simulink model "QuadcopterModel"  (R2018a)
settings: Solver=ode1  StartTime=0.0  StopTime=10.0  FixedStep=T  RelTol=1e-3  EnableMultiTasking=on
undefined symbols (not defined in the file): g, I, I_add, I_add_time, K, L, m, m_add, m_add_time, omega0, Phi0, Psi0, rho_ge, Rp, T_add, T_add_time, Theta0, V0, X0, Xmax, Xmin, Zg
libraries: UAV_Control x3
settings Model: Creator=ahmad  LastModifiedBy=Ahmad
settings OptimizationCC: LifeSpan=inf
settings DebuggingCC: SFUnexpectedBacktrackingDiag=warning  SFNoUnconditionalDefaultTransitionDiag=warning  SFExecutionAtInitializationDiag=none
settings CodeAppCC: StateflowObjectComments=on
settings GRTTargetCC: TargetLangStandard=C89/C90 (ANSI)  GeneratePreprocessorConditionals=Disable all
settings ConfigComp: CovMetricSettings=dw  CovHtmlReporting=on  CovSaveCumulativeToWorkspaceVar=on  CovSaveSingleToWorkspaceVar=on  CovExternalEMLEnable=off

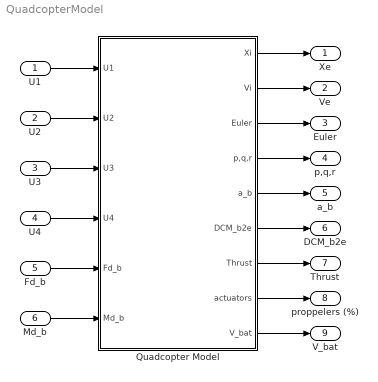
== system QuadcopterModel ==
  U1 : Inport
  U2 : Inport  Port=2
  U3 : Inport  Port=3
  U4 : Inport  Port=4
  Fd_b : Inport  Port=5
  Md_b : Inport  Port=6
  Quadcopter Model : Subsystem  mask(QuadcopterModel){}
      mask Display:
      | port_label('input',1,'U1','texmode','on')
      | port_label('input',2,'U2','texmode','on')
      | port_label('input',3,'U3','texmode','on')
      | port_label('input',4,'U4','texmode','on')
      | port_label('input',5,'Fd_b','texmode','on')
      | port_label('input',6,'Md_b','texmode','on')
      | 
      | port_label('output',1,'Xe (m)','texmode','on')
      | port_label('output',2,'Ve (m/s)','texmode','on')
      | port_label('output',3,'\phi \theta \psi (rad/s)','texmode','on')
      | port_label('output',4,'p,q,r (rad/s^2)','texmode','on')
      | port_label('output',5,'a_b (m/s^2)','texmode','on')
      | port_label('output',6,'DCM_{b2e}','texmode','on')
      | port_label('output',7,'Thrust (N)','texmode','on')
      | port_label('output',8,'proppelers (%)','texmode','on')
      | port_label('output',9,'V_{bat}','texmode','on')
  Xe : Outport
  Ve : Outport  Port=2
  "Euler " : Outport  Port=3
  p,q,r : Outport  Port=4
  a_b : Outport  Port=5
  DCM_b2e : Outport  Port=6
  Thrust : Outport  Port=7
  proppelers (%) : Outport  Port=8
  V_bat : Outport  Port=9
  wires:
  U1/1 -> Quadcopter Model/1(U1)
  U2/1 -> Quadcopter Model/2(U2)
  U3/1 -> Quadcopter Model/3(U3)
  Quadcopter Model/1(Xi) -> Xe/1
  Quadcopter Model/2(Vi) -> Ve/1
  Quadcopter Model/3("Euler ") -> "Euler "/1
  Quadcopter Model/4(p,q,r) -> p,q,r/1
  U4/1 -> Quadcopter Model/4(U4)
  Quadcopter Model/7(Thrust) -> Thrust/1
  Fd_b/1 -> Quadcopter Model/5(Fd_b)
  Quadcopter Model/8(actuators) -> proppelers (%)/1
  Quadcopter Model/6(DCM_b2e) -> DCM_b2e/1
  Quadcopter Model/5(a_b) -> a_b/1
  Md_b/1 -> Quadcopter Model/6(Md_b)
  Quadcopter Model/9(V_bat) -> V_bat/1

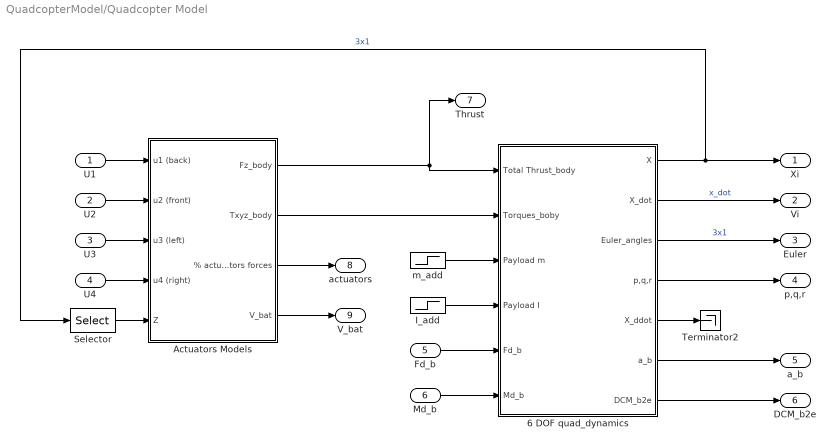
== system QuadcopterModel/Quadcopter Model ==
  U1 : Inport
  U2 : Inport  Port=2
  U3 : Inport  Port=3
  U4 : Inport  Port=4
  Fd_b : Inport  Port=5
  Md_b : Inport  Port=6
  6 DOF quad_dynamics : Subsystem
  Actuators Models : Subsystem
  I_add : Step  Time=I_add_time  After=I_add  SampleTime=0
  Selector : Selector  InputPortWidth=3  IndexOptions=Index vector (dialog)  Indices=3  OutputSizes=1
  Terminator2 : Terminator
  m_add : Step  Time=m_add_time  After=m_add  SampleTime=0
  Xi : Outport
  Vi : Outport  Port=2
  "Euler " : Outport  Port=3
  p,q,r : Outport  Port=4
  a_b : Outport  Port=5
  DCM_b2e : Outport  Port=6
  Thrust : Outport  Port=7
  actuators : Outport  Port=8
  V_bat : Outport  Port=9
  wires:
  6 DOF quad_dynamics/3(Euler_angles) -> "Euler "/1  "3x1"
  6 DOF quad_dynamics/2(X_dot) -> Vi/1  "x_dot"
  6 DOF quad_dynamics/4(p,q,r) -> p,q,r/1
  U2/1 -> Actuators Models/2(u2 (front))
  U3/1 -> Actuators Models/3(u3 (left))
  U4/1 -> Actuators Models/4(u4 (right))
  Actuators Models/3(% actuators forces) -> actuators/1
  6 DOF quad_dynamics/6(a_b) -> a_b/1
  6 DOF quad_dynamics/1(X) -> Selector/1, Xi/1  "3x1"
  U1/1 -> Actuators Models/1(u1 (back))
  Actuators Models/1(Fz_body) -> 6 DOF quad_dynamics/1("Total Thrust_body "), Thrust/1
  Actuators Models/2(Txyz_body) -> 6 DOF quad_dynamics/2(Torques_boby)
  Fd_b/1 -> 6 DOF quad_dynamics/5(Fd_b)
  6 DOF quad_dynamics/7(DCM_b2e) -> DCM_b2e/1
  6 DOF quad_dynamics/5(X_ddot) -> Terminator2/1
  m_add/1 -> 6 DOF quad_dynamics/3(Payload m)
  I_add/1 -> 6 DOF quad_dynamics/4("Payload I ")
  Md_b/1 -> 6 DOF quad_dynamics/6(Md_b)
  Selector/1 -> Actuators Models/5(Z)
  Actuators Models/4(V_bat) -> V_bat/1

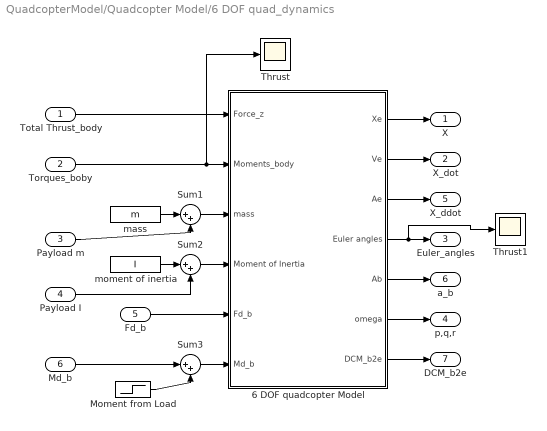
== system QuadcopterModel/Quadcopter Model/6 DOF quad_dynamics ==
  "Total Thrust_body " : Inport
  Torques_boby : Inport  Port=2
  Payload m : Inport  Port=3
  "Payload I " : Inport  Port=4
  Fd_b : Inport  Port=5  PortDimensions=3
  Md_b : Inport  Port=6  PortDimensions=3
  6 DOF quadcopter Model : Subsystem  mask(6DOF rigid body){h0=Zg, X0=X0, V0=V0, Euler0=[Phi0 Theta0 Psi0], omega0=omega0, X_min=Xmin, X_max=Xmax, g=g}
      mask prompts: h0 "Ground height:"; X0 "Initial Position:"; V0 "Initial Velocity:"; Euler0 "Initial euler angles:"; omega0 "Initial angular velocites:"; X_min "Position Lower Bound:"; X_max "Position Upper Bound:"; g "Gravity:"
      mask help: Determines the rotational motion of a 6DOF rigid body.
      mask Help:
      | alpha=Mb/I - omega x omega
      | omega=alpha_dot
      | Euler=omega_dot
      | 
      | a_b = Fb/m-omega x V_b
      | a_e = R_b2e*a_b
      | V_e = a_e_dot
      | Xe = V_e_dot
      mask Display:
      | port_label('input',1,'Fz (N)','texmode','on')
      | port_label('input',2,'M_b (N.m)','texmode','on')
      | port_label('input',3,'m (kg)','texmode','on')
      | port_label('input',4,'I (kg/m^2)','texmode','on')
      | port_label('input',5,'Fd_b (N)','texmode','on')
      | port_label('input',6,'Md_b (N.m)','texmode','on')
      | 
      | 
      | port_label('output',1,'X_e (m)','texmode','on')
      | port_label('output',2,'V_e (m/s)','texmode','on')
      | port_label('output',3,'a_e (m/s^2)','texmode','on')
      | port_label('output',4,'\phi,\theta,\psi (rad)','texmode','on')
      | port_label('output',5,'a_b (m/s^2)','texmode','on')
      | port_label('output',6,'\omega (rad/s)','texmode','on')
      | port_label('output',7,'DCM_{b2e}','texmode','on')
  Moment from Load : Step  Time=T_add_time  After=T_add  SampleTime=0
  Sum1 : Sum  Inputs=|++
  Sum2 : Sum  Inputs=|++
  Sum3 : Sum  Inputs=|++
  Thrust : Scope
  Thrust1 : Scope
  mass : Constant  Value=m
  moment of inertia : Constant  Value=I
  X : Outport
  X_dot : Outport  Port=2
  Euler_angles : Outport  Port=3
  p,q,r : Outport  Port=4
  X_ddot : Outport  Port=5
  a_b : Outport  Port=6
  DCM_b2e : Outport  Port=7
  wires:
  Payload m/1 -> Sum1/2
  mass/1 -> Sum1/1
  "Total Thrust_body "/1 -> 6 DOF quadcopter Model/1(Force_z)
  Torques_boby/1 -> 6 DOF quadcopter Model/2(Moments_body), Thrust/1
  Sum2/1 -> 6 DOF quadcopter Model/4(Moment of Inertia)
  Sum1/1 -> 6 DOF quadcopter Model/3(mass)
  6 DOF quadcopter Model/1(Xe) -> X/1
  6 DOF quadcopter Model/2(Ve) -> X_dot/1
  6 DOF quadcopter Model/3(Ae) -> X_ddot/1
  6 DOF quadcopter Model/4(Euler angles) -> Thrust1/1, Euler_angles/1
  moment of inertia/1 -> Sum2/1
  "Payload I "/1 -> Sum2/2
  6 DOF quadcopter Model/7(DCM_b2e) -> DCM_b2e/1
  6 DOF quadcopter Model/6(omega) -> p,q,r/1
  6 DOF quadcopter Model/5(Ab) -> a_b/1
  Fd_b/1 -> 6 DOF quadcopter Model/5(Fd_b)
  Sum3/1 -> 6 DOF quadcopter Model/6(Md_b)
  Md_b/1 -> Sum3/1
  Moment from Load/1 -> Sum3/2

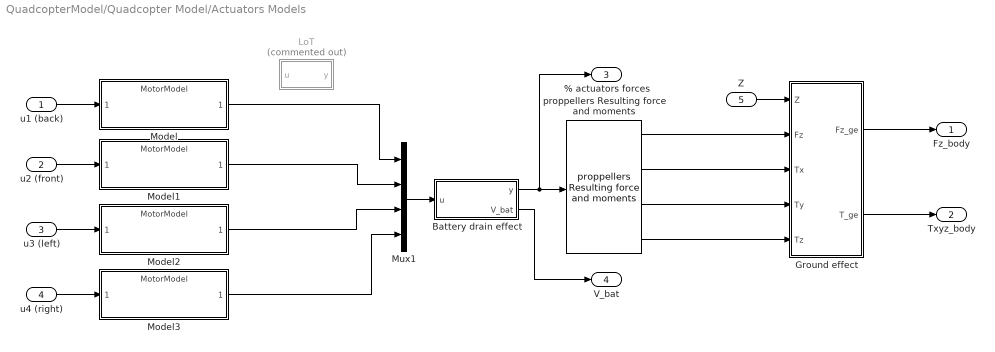
== system QuadcopterModel/Quadcopter Model/Actuators Models ==
  u1 (back) : Inport
  u2 (front) : Inport  Port=2
  u3 (left) : Inport  Port=3
  u4 (right) : Inport  Port=4
  Z : Inport  Port=5
  Battery drain effect : Subsystem
  Ground effect : Subsystem
  LoT : Subsystem  Commented=on
  Model{,1..3} (4 alike) : ModelReference  ModelNameDialog=MotorModel.slx  SimulationMode=Normal  ModelReferenceVersion=1.12
  Mux1 : Mux
  proppellers Resulting force and moments : UAV_Control/proppellers Resulting force and moments  K=K  Ky=Ky  L=L
      settings: SourceProductName=UAV_Control
  Fz_body : Outport
  Txyz_body : Outport  Port=2
  % actuators forces : Outport  Port=3
  V_bat : Outport  Port=4
  wires:
  u1 (back)/1 -> Model/1
  u2 (front)/1 -> Model1/1
  u4 (right)/1 -> Model3/1
  Mux1/1 -> Battery drain effect/1(u)
  Model3/1 -> Mux1/4
  u3 (left)/1 -> Model2/1
  Model/1 -> Mux1/1
  Model2/1 -> Mux1/3
  Model1/1 -> Mux1/2
  Z/1 -> Ground effect/1(Z)
  proppellers Resulting force and moments/1 -> Ground effect/2(Fz)
  proppellers Resulting force and moments/2 -> Ground effect/3(Tx)
  proppellers Resulting force and moments/3 -> Ground effect/4(Ty)
  proppellers Resulting force and moments/4 -> Ground effect/5(Tz)
  Ground effect/1(Fz_ge) -> Fz_body/1
  Ground effect/2(T_ge) -> Txyz_body/1
  Battery drain effect/1(y) -> proppellers Resulting force and moments/1, % actuators forces/1
  Battery drain effect/2(V_bat) -> V_bat/1

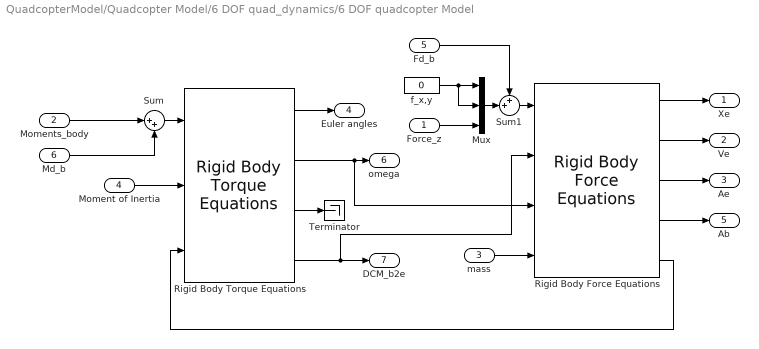
== system QuadcopterModel/Quadcopter Model/6 DOF quad_dynamics/6 DOF quadcopter Model ==
  Force_z : Inport
  Moments_body : Inport  Port=2
  mass : Inport  Port=3
  Moment of Inertia : Inport  Port=4
  Fd_b : Inport  Port=5
  Md_b : Inport  Port=6
  Mux : Mux  Inputs=3
  Rigid Body Force Equations : UAV_Control/Rigid Body Force Equations  g=g  h0=Zg  X0=X0  X_min=Xmin  X_max=Xmax  V0=V0
      settings: SourceProductName=UAV_Control
  "Rigid Body Torque Equations " : UAV_Control/Rigid Body Torque Equations   Euler0=[Phi0 Theta0 Psi0]  omega0=omega0
      settings: SourceProductName=UAV_Control
  Sum : Sum  Inputs=|++
  Sum1 : Sum  Inputs=++|
  Terminator : Terminator
  f_x,y : Constant  Value=0
  Xe : Outport
  Ve : Outport  Port=2
  Ae : Outport  Port=3
  Euler angles : Outport  Port=4
  Ab : Outport  Port=5
  omega : Outport  Port=6
  DCM_b2e : Outport  Port=7
  wires:
  Rigid Body Force Equations/1 -> Xe/1
  "Rigid Body Torque Equations "/3 -> Terminator/1
  "Rigid Body Torque Equations "/2 -> Rigid Body Force Equations/3, omega/1
  "Rigid Body Torque Equations "/1 -> Euler angles/1
  Rigid Body Force Equations/3 -> Ae/1
  Rigid Body Force Equations/2 -> Ve/1
  mass/1 -> Rigid Body Force Equations/4
  Moment of Inertia/1 -> "Rigid Body Torque Equations "/2
  "Rigid Body Torque Equations "/4 -> Rigid Body Force Equations/2, DCM_b2e/1
  Rigid Body Force Equations/4 -> Ab/1
  Sum/1 -> "Rigid Body Torque Equations "/1
  Moments_body/1 -> Sum/1
  Md_b/1 -> Sum/2
  Rigid Body Force Equations/5 -> "Rigid Body Torque Equations "/3
  Sum1/1 -> Rigid Body Force Equations/1
  f_x,y/1 -> Mux/2, Mux/1
  Force_z/1 -> Mux/3
  Mux/1 -> Sum1/2
  Fd_b/1 -> Sum1/1

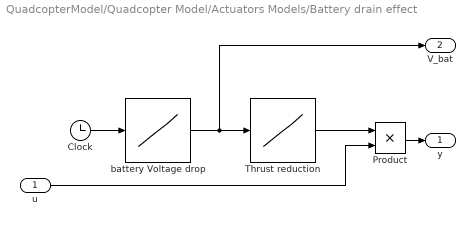
== system QuadcopterModel/Quadcopter Model/Actuators Models/Battery drain effect ==
  u : Inport
  Clock : Clock
  Product : Product
  Thrust reduction : Lookup_n-D  NumberOfTableDimensions=1  BreakpointsForDimension1=[10 12]  Table=[0.8 1]  InternalRulePriority=Speed  RndMeth=Simplest  InputSameDT=on
  battery Voltage drop : Lookup_n-D  NumberOfTableDimensions=1  BreakpointsForDimension1=[0 360]  Table=[12 10]  InternalRulePriority=Speed  RndMeth=Simplest  InputSameDT=on
  y : Outport
  V_bat : Outport  Port=2
  wires:
  u/1 -> Product/2
  Clock/1 -> battery Voltage drop/1
  Thrust reduction/1 -> Product/1
  Product/1 -> y/1
  battery Voltage drop/1 -> V_bat/1, Thrust reduction/1

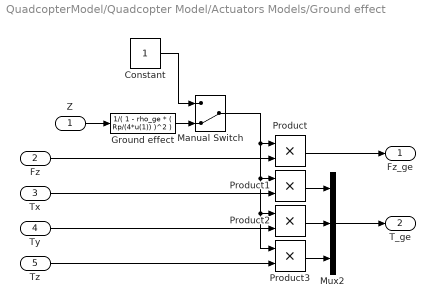
== system QuadcopterModel/Quadcopter Model/Actuators Models/Ground effect ==
  Z : Inport
  Fz : Inport  Port=2
  Tx : Inport  Port=3
  Ty : Inport  Port=4
  Tz : Inport  Port=5
  Constant : Constant
  Ground effect : Fcn  Expr=1/( 1 - rho_ge * ( Rp/(4*u(1)) )^2 )
  Manual Switch : ManualSwitch  CurrentSetting=0
  Mux2 : Mux  Inputs=3
  Product{,1..3} (4 alike) : Product
  Fz_ge : Outport
  T_ge : Outport  Port=2
  wires:
  Manual Switch/1 -> Product3/1, Product2/1, Product1/1, Product/1
  Ty/1 -> Product2/2
  Product2/1 -> Mux2/2
  Z/1 -> Ground effect/1
  Tz/1 -> Product3/2
  Product/1 -> Fz_ge/1
  Fz/1 -> Product/2
  Product3/1 -> Mux2/3
  Product1/1 -> Mux2/1
  Mux2/1 -> T_ge/1
  Tx/1 -> Product1/2
  Ground effect/1 -> Manual Switch/2
  Constant/1 -> Manual Switch/1

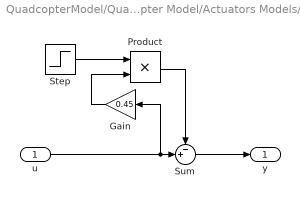
== system QuadcopterModel/Quadcopter Model/Actuators Models/LoT ==
  u : Inport
  Gain : Gain  Gain=0.45
  Product : Product
  Step : Step  Time=50  SampleTime=0
  Sum : Sum  Inputs=-+|
  y : Outport
  wires:
  Step/1 -> Product/1
  Product/1 -> Sum/1
  u/1 -> Gain/1, Sum/2
  Sum/1 -> y/1
  Gain/1 -> Product/2
